simulink model "einfacher_Prozess_Zust_Beob"  (Simulink 7.5)
settings: Solver=ode45  StartTime=0.0  StopTime=10.0  RelTol=1e-3
values from neighbouring files (symbols this model uses):
  KV = KV'    [Reglerauslegung.m]    (also in Test_Reglerauslegung.m; auslegung.m)
undefined symbols (not defined in the file or in its folder): KB1, KB2, KB3, KR1, KR2, KR3, MU3
settings Model: Creator=Mattse  LastModifiedBy=Mattse
settings DebuggingCC: FcnCallInpInsideContextMsg=Enable All

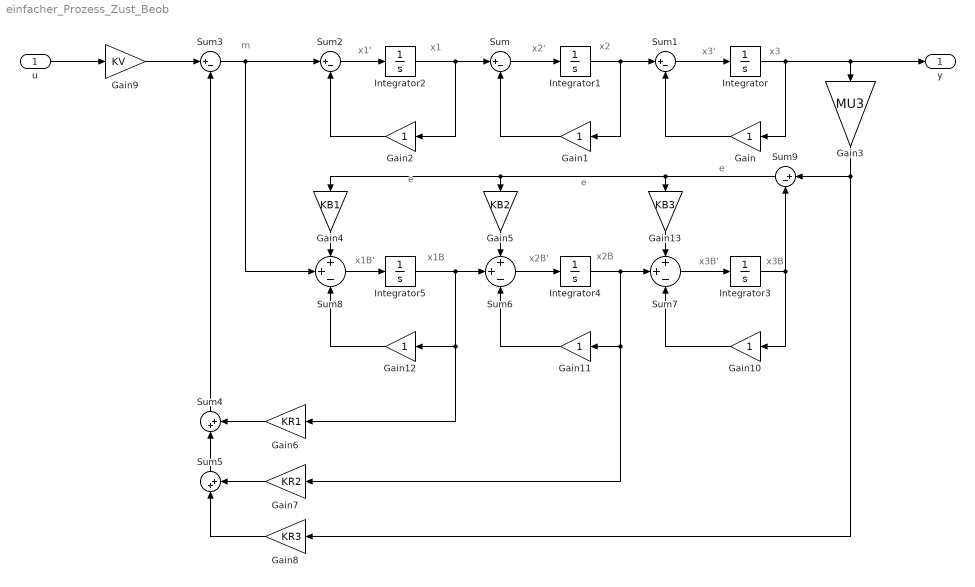
== system einfacher_Prozess_Zust_Beob ==
  note: x1'
  note: x1
  note: x2'
  note: x2
  note: x3'
  note: x3
  note: x1B'
  note: x1B
  note: x2B'
  note: x2B
  note: x3B'
  note: x3B
  note: m
  note: e
  note: e
  note: e
  u : Inport
  Gain{,1..2,10..12} (6 alike) : Gain
  Gain13 : Gain  Gain=KB3
  Gain3 : Gain  Gain=MU3
  Gain4 : Gain  Gain=KB1
  Gain5 : Gain  Gain=KB2
  Gain6 : Gain  Gain=KR1
  Gain7 : Gain  Gain=KR2
  Gain8 : Gain  Gain=KR3
  Gain9 : Gain  Gain=KV
  Integrator{,1..5} (6 alike) : Integrator
  Sum{,1..3,9} (5 alike) : Sum  Inputs=|+-
  Sum4 : Sum  Inputs=|++
  Sum5 : Sum  Inputs=|++
  Sum6 : Sum  Inputs=++-
  Sum7 : Sum  Inputs=++-
  Sum8 : Sum  Inputs=++-
  y : Outport
  wires:
  Integrator1/1 -> Sum1/1, Gain1/1
  Sum1/1 -> Integrator/1
  Sum/1 -> Integrator1/1
  Integrator2/1 -> Sum/1, Gain2/1
  Sum2/1 -> Integrator2/1
  Integrator/1 -> Gain/1, y/1, Gain3/1
  Gain/1 -> Sum1/2
  Gain1/1 -> Sum/2
  Gain2/1 -> Sum2/2
  Sum3/1 -> Sum2/1, Sum8/2
  Gain6/1 -> Sum4/2
  Gain8/1 -> Sum5/1
  Gain7/1 -> Sum5/2
  Sum5/1 -> Sum4/1
  Sum4/1 -> Sum3/2
  u/1 -> Gain9/1
  Gain9/1 -> Sum3/1
  Integrator4/1 -> Gain11/1, Gain7/1, Sum7/2
  Sum7/1 -> Integrator3/1
  Integrator5/1 -> Gain12/1, Gain6/1, Sum6/2
  Sum8/1 -> Integrator5/1
  Integrator3/1 -> Sum9/2, Gain10/1
  Gain10/1 -> Sum7/3
  Gain12/1 -> Sum8/3
  Gain11/1 -> Sum6/3
  Sum6/1 -> Integrator4/1
  Gain3/1 -> Sum9/1, Gain8/1
  Gain4/1 -> Sum8/1
  Sum9/1 -> Gain4/1, Gain5/1, Gain13/1
  Gain5/1 -> Sum6/1
  Gain13/1 -> Sum7/1
